simulink model "battery_convertidor_ac_dc_44"  (R2024b)
settings: Solver=FixedStepAuto  StartTime=0.0  StopTime=751  FixedStep=1e-5  RelTol=1e-3
InitFcn:
  | Tint = 1e-5;
  | Ts = 10*Tint;
values from neighbouring files (symbols this model uses):
  C1_filter = 20e-6    (= 2e-05)    [parametros_generales.m]
  I_control = 1    [parametros_generales.m]
  I_control_bat = 5    [parametros_generales.m]
  L_converter = 20e-3    (= 0.02)    [parametros_generales.m]
  Lbat_converter = 1e-5    (= 1e-05)    [parametros_generales.m]
  load_dc = 1000*1000/5    (= 200000)    [parametros_generales.m]
  P_control = 0.01    [parametros_generales.m]
  P_control_bat = 0.7    [parametros_generales.m]
  R = 0.5    [parametros_generales.m]
  R_filter = 0.5    [parametros_generales.m]
  rated_capacitance = 62.5/8    (= 7.8125)    [parametros_generales.m]
  rated_voltage = 144*8    (= 1152)    [parametros_generales.m]
  sample_time_control = 4e-4    (= 0.0004)    [parametros_generales.m]
  voltage_dc_source = 1000    [parametros_generales.m]
undefined symbols (not defined in the file or in its folder): Ion, Lithium
libraries: spsIGBTDiodeLib x24, spsCurrentMeasurementLib x23, spsSeriesRLCBranchLib x20, spsVoltageMeasurementLib x14, dspstat3 x8, spsThreePhaseVIMeasurementLib x8, simulink x7, spsPower3phInstantaneousLib x6, slpidlib x3, spsBatteryLib x2, spsVariableCapacitorLib x1, spsVariableResistorLib x1
(part 1 of 2)
settings Model: Creator=DGY  LastModifiedBy=dagua
settings DataIOCC: SignalLogging=off  DSMLogging=off  ReturnWorkspaceOutputs=off
settings DebuggingCC: UnconnectedInputMsg=warning  UnconnectedOutputMsg=warning  UnconnectedLineMsg=warning
settings ModelReferenceCC: EnableRefExpFcnMdlSchedulingChecks=on
settings RTWCC: GPUComputeCapability=3.5  DLArmComputeVersion=19.05

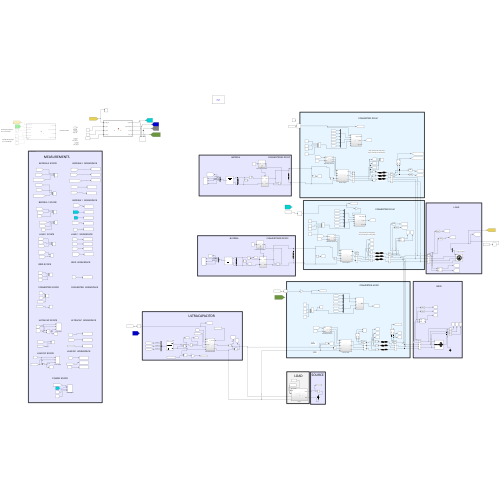
[thumbnail: Simulink's stored preview of the top-level diagram]
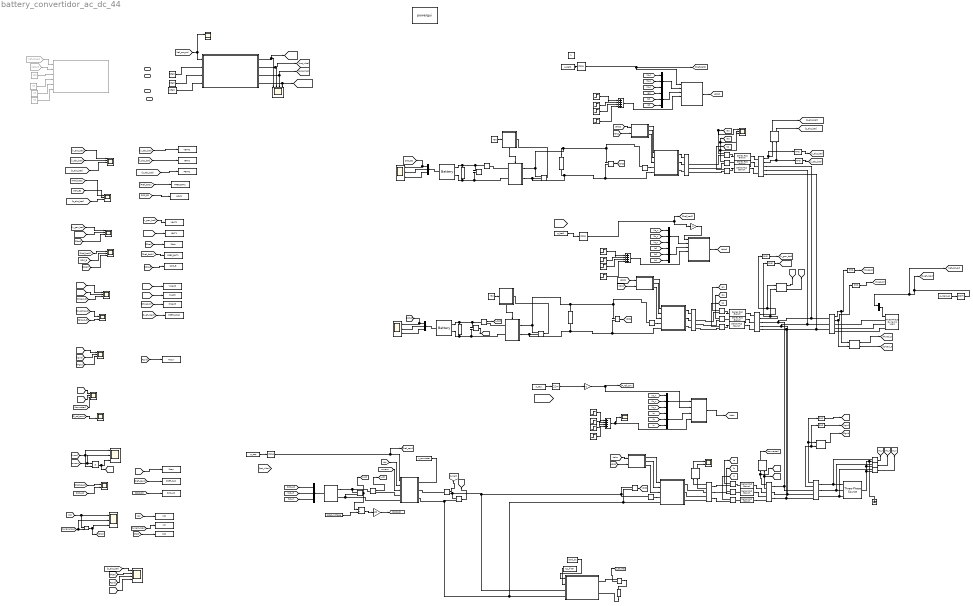
== system battery_convertidor_ac_dc_44 ==
  note: carga en estrella
  note: raiz(3)*Ip/raiz(2)*Vph*raiz(3)/raiz(2)
  note: potencias manuales
  note: i1
  note: Visualización
  note: i2
  note: BATERIA
  note: CONVERTIDOR DC/DC
  note: CONVERTER DC/AC
  note: CONVERTER AC/DC
  note: DC+
  note: DC-
  note: MEASUREMENTS
  note: porcentaje de energia que va a ir a la carga AC
  note: porcentaje de energia que va a ir a la carga DC
  note: raiz(3)*102/raiz(2)*327*raiz(3)/raiz(2)
  note: SOURCE
  note: 35kw
  note: ULTRACAPACITOR
  note: 7s1p
  note: LOAD
  note: 1154
  note: raiz(3)*Ip/raiz(2)*Vph*raiz(3)/raiz(2)
  note: CONVERTIDOR DC/DC
  note: BATERIA
  note: raiz(3)*102/raiz(2)*327*raiz(3)/raiz(2)
  note: CONVERTER DC/AC
  note: BATERIA 2 SCOPE
  note: BATERIA 2 WORKSPACE
  note: BATERIA 1 SCOPE
  note: BATERIA 1 WORKSPACE
  note: GRID SCOPE
  note: GRID WORKSPACE
  note: LOAD
  note: GRID
  note: LOAD 1 WORKSPACE
  note: LOAD 1 SCOPE
  note: ULTRACAP WORKSPACE
  note: ULTRACAP SCOPE
  note: CONVERTER SCOPE
  note: CONVERTER WORKSPACE
  note: LOAD DC WORKSPACE
  note: LOAD DC SCOPE
  note: POWER SCOPE
  Pref_Bat : Inport
  Pref_Ultr : Inport  Port=2
  Pref_smes : Inport  Port=3
  Pref_ac_dc : Inport  Port=4
  Battery : spsBatteryLib/Battery  BatType=Lithium-Ion  NomV=Nominal_voltage  NomQ=Rated_capacity  SOC=initial_state_of_charge  Batt_Tr=battery_time  PresetModel=on  MaxQ=1000  MinV=384  FullV=595.9614  Dis_rate=434.7826  R=0.00512  Normal_OP=904.3478  expZone="[553.1576      49.13043]"
      settings: LibrarySourceBlock=electricdrivelib/Extra Sources/Battery
  Battery1 : spsBatteryLib/Battery  BatType=Lithium-Ion  NomV=Nominal_voltage  NomQ=Rated_capacity  SOC=initial_state_of_charge  Batt_Tr=battery_time  PresetModel=on  MaxQ=1000  MinV=384  FullV=595.9614  Dis_rate=434.7826  R=0.00512  Normal_OP=904.3478  expZone="[553.1576      49.13043]"
      settings: LibrarySourceBlock=electricdrivelib/Extra Sources/Battery
  Bus Selector : BusSelector  OutputSignals=SOC (%),Current (A),Voltage (V)
  Bus Selector1 : BusSelector  OutputSignals=SOC (%),Current (A),Voltage (V)
  Bus Selector2 : BusSelector  OutputSignals=SOC %,Voltage V,Current I
  Carga : Subsystem
  Constant : Constant
  Constant1 : Constant  Value=C1_filter
  Constant10 : Constant  Value=25e3
  Constant13 : Constant  Value=25e3
  Constant15 : Constant  Value=83e3
  Constant16 : Constant  Commented=on  Value=33
  Constant17 : Constant  Commented=on  Value=100
  Constant2 : Constant  Value=750
  Constant3 : Constant  Value=750
  Constant4 : Constant  Value=load_dc
  Constant5 : Constant  Value=rated_voltage
  Constant6 : Constant  Value=L_converter
  Constant8 : Constant  Commented=on  Value=33
  Constant9 : Constant  Commented=on  Value=33
  Control del convertidor1 : Subsystem
      settings: PortSchema="{\"entries\":[{\"content\":{\"sides\":[{\"content\":{\"connectorIds\":[\"In1\"]},\"type\":\"ConnectorPlacement.EquallySpacedRectSide\",\"uuid\":\"952f4d9f-85a3-4809-ab80-f95b4e630059\"},{\"content\":{\"connectorIds\":[\"In2\"],\"side\":\"RIGHT\"},\"type\":\"ConnectorPlacement.EquallySpacedRectSide\",\"uuid\":\"24c0a236-3f22-4c40-86cc-925551a19bc9\"},{\"content\":{\"side\":\"TOP\"},\"type\":\"ConnectorPlacement.EquallySpacedRectSide\",\"uuid\":\"1a366aec-943f-41ae-ba47-6c948c084703\"},{\"content\":{\"connectorIds\":[\"Out1\"],\"side\":\"BOTTOM\"},\"type\":\"ConnectorPlacement.EquallySpacedRectSide\",\"uuid\":\"781da9ee-8b6b-417d-a56c-b699191914ae\"}]},\"type\":\"ConnectorPlacement.EquallySpacedConnector\",\"uuid\":\"c6d9e875-0dde-4ffd-9bd0-64114f723d5e\"}],\"packageUris\":[\"http://schema.mathworks.com/mf0/Connector/R2020b\"],\"version\":\"1.0\"}"
  Control del convertidor2 : Subsystem
      settings: PortSchema="{\"entries\":[{\"content\":{\"sides\":[{\"content\":{\"connectorIds\":[\"In1\"]},\"type\":\"ConnectorPlacement.EquallySpacedRectSide\",\"uuid\":\"952f4d9f-85a3-4809-ab80-f95b4e630059\"},{\"content\":{\"connectorIds\":[\"In2\"],\"side\":\"RIGHT\"},\"type\":\"ConnectorPlacement.EquallySpacedRectSide\",\"uuid\":\"24c0a236-3f22-4c40-86cc-925551a19bc9\"},{\"content\":{\"side\":\"TOP\"},\"type\":\"ConnectorPlacement.EquallySpacedRectSide\",\"uuid\":\"1a366aec-943f-41ae-ba47-6c948c084703\"},{\"content\":{\"connectorIds\":[\"Out1\"],\"side\":\"BOTTOM\"},\"type\":\"ConnectorPlacement.EquallySpacedRectSide\",\"uuid\":\"781da9ee-8b6b-417d-a56c-b699191914ae\"}]},\"type\":\"ConnectorPlacement.EquallySpacedConnector\",\"uuid\":\"c6d9e875-0dde-4ffd-9bd0-64114f723d5e\"}],\"packageUris\":[\"http://schema.mathworks.com/mf0/Connector/R2020b\"],\"version\":\"1.0\"}"
  Current Measurement{,1..16} (17 alike) : spsCurrentMeasurementLib/Current Measurement  PhasorSimulation=off  OutputType=Complex  PSBequivalent=0
  DC Voltage Source1 : spsDCVoltageSourceLib/DC Voltage Source  Amplitude=voltage_dc_source  Measurements=None
  Divide1 : Product  Inputs=*/
  From Workspace : FromWorkspace  VariableName=p_bat1
  From Workspace1 : FromWorkspace  VariableName=p_cap
  From Workspace2 : FromWorkspace  VariableName=p_cap
  From Workspace3 : FromWorkspace  VariableName=p_load_ac
  From Workspace4 : FromWorkspace  VariableName=p_bat2
  From43 : From  Commented=on  GotoTag=ref_pot_ac
  From55 : From  Commented=on  GotoTag=refpot
  Gain1 : Gain  Gain=-1
  Gain2 : Gain  Gain=-1
  Gain3 : Gain  Gain=100
  Ground : spsGroundLib/Ground  LConnTagsString=a
  MATLAB Function : MATLAB Function  Commented=on  TreatAsAtomicUnit=on
  MATLAB Function1 : MATLAB Function  TreatAsAtomicUnit=on
  Modulación puente H1 : Subsystem
  Modulación puente H2 : Subsystem
  Modulación puente H3 : Subsystem
  Mux{1..4,12..13} (6 alike) : Mux  Inputs=3
  Mux17 : Mux  Inputs=2
  Power (3ph, Instantaneous){,2..5,7} (6 alike) : spsPower3phInstantaneousLib/Power (3ph, Instantaneous)
  Product2 : Product
  Product4 : Product
  Puente H 3pha : Subsystem
  Puente H 3pha1 : Subsystem
  Puente H 3pha2 : Subsystem
  RMS{,1..7} (8 alike) : dspstat3/RMS  run=off  directionMode=Each column  dimension=1  InputProcessing=Columns as channels (frame based)  reset_popup=None
  Scope{,1,15,21,41} (5 alike) : Scope  NumInputPorts=2
  Scope{2..3,5,7..8,12,23} (7 alike) : Scope  NumInputPorts=3
  Scope{6,14,19..20} (4 alike) : Scope  NumInputPorts=4
  Scope9 : Scope
  Series RLC Branch{1..4,7..8,11..13} (9 alike) : spsSeriesRLCBranchLib/Series RLC Branch  LConnTagsString=__new0  RConnTagsString=__new0  BranchType=RL  Resistance=0.2  Inductance=5e-3  SetiL0=off  InitialCurrent=0  Capacitance=1e-6  Setx0=off  InitialVoltage=0  Measurements=None
  Series RLC Branch10 : spsSeriesRLCBranchLib/Series RLC Branch  LConnTagsString=__new0  RConnTagsString=__new0  BranchType=RC  Resistance=0.001  Inductance=1e-3  SetiL0=off  InitialCurrent=0  Capacitance=1e-2  Setx0=on  InitialVoltage=512  Measurements=None
  Series RLC Branch5 : spsSeriesRLCBranchLib/Series RLC Branch  LConnTagsString=__new0  RConnTagsString=__new0  BranchType=C  Resistance=0.2  Inductance=1e-3  SetiL0=off  InitialCurrent=0  Capacitance=0.15  Setx0=on  InitialVoltage=600  Measurements=None
  Series RLC Branch6 : spsSeriesRLCBranchLib/Series RLC Branch  LConnTagsString=__new0  RConnTagsString=__new0  BranchType=RC  Resistance=0.001  Inductance=1e-3  SetiL0=off  InitialCurrent=0  Capacitance=1e-2  Setx0=on  InitialVoltage=512  Measurements=None
  Series RLC Branch9 : spsSeriesRLCBranchLib/Series RLC Branch  LConnTagsString=__new0  RConnTagsString=__new0  BranchType=C  Resistance=0.2  Inductance=1e-3  SetiL0=off  InitialCurrent=0  Capacitance=0.15  Setx0=on  InitialVoltage=600  Measurements=None
  Step12 : Step  Time=0.1  Before=-1.5e3  After=-2e3  SampleTime=0
  Step16 : Step  Time=0.2  After=-1e3  SampleTime=0
  Step17 : Step  Time=0.1  Before=-1.5e3  After=-2e3  SampleTime=0
  Step18 : Step  Time=0.2  After=-1e3  SampleTime=0
  Step19 : Step  Time=0.3  After=-1e3  SampleTime=0
  Step20 : Step  Time=0.4  After=-1e3  SampleTime=0
  Step21 : Step  Time=0.3  After=-1e3  SampleTime=0
  Step22 : Step  Time=0.4  After=-1e3  SampleTime=0
  Step6 : Step  Time=0.15  Before=1.5e3  After=2e3  SampleTime=0
  Step7 : Step  Time=0.3  After=1e3  SampleTime=0
  Step8 : Step  Time=0.45  After=1e3  SampleTime=0
  Step9 : Step  After=1e3  SampleTime=0
  "Subs switched model " : Subsystem
      settings: PortSchema="{\"entries\":[{\"content\":{\"sides\":[{\"content\":{\"connectorIds\":[\"In1\",\"In2\",\"In3\",\"LConn1\",\"LConn2\"]},\"type\":\"ConnectorPlacement.EquallySpacedRectSide\",\"uuid\":\"c251221c-47f6-421c-a2d7-5bbfba4f112f\"},{\"content\":{\"connectorIds\":[\"In4\",\"RConn1\",\"RConn2\"],\"side\":\"RIGHT\"},\"type\":\"ConnectorPlacement.EquallySpacedRectSide\",\"uuid\":\"04a66283-5a4b-4f04-b1e9-633aa9198ece\"},{\"content\":{\"side\":\"TOP\"},\"type\":\"ConnectorPlacement.EquallySpacedRectSide\",\"uuid\":\"bb199fa0-295e-40b6-9755-cc304ea24fe5\"}]},\"type\":\"ConnectorPlacement.EquallySpacedConnector\",\"uuid\":\"0b09f002-5912-488f-a17f-ab220b7325f4\"}],\"packageUris\":[\"http://schema.mathworks.com/mf0/Connector/R2020b\"],\"version\":\"1.0\"}"
  Subsystem : Subsystem
  Subsystem1 : Subsystem
  Subsystem2 : Subsystem
  Subsystem3 : Subsystem
      settings: PortSchema="{\"entries\":[{\"content\":{\"sides\":[{\"content\":{\"connectorIds\":[\"LConn1\",\"LConn2\"]},\"type\":\"ConnectorPlacement.EquallySpacedRectSide\",\"uuid\":\"7a980847-0fd3-4a52-ae22-59cd2a1ed559\"},{\"content\":{\"connectorIds\":[\"RConn1\",\"RConn2\"],\"side\":\"RIGHT\"},\"type\":\"ConnectorPlacement.EquallySpacedRectSide\",\"uuid\":\"85effeeb-73a6-4b0a-b51b-5eb0082317ff\"},{\"content\":{\"connectorIds\":[\"In1\"],\"side\":\"TOP\"},\"type\":\"ConnectorPlacement.EquallySpacedRectSide\",\"uuid\":\"eb55fae0-79ad-414f-ab96-49c332138803\"},{\"content\":{\"side\":\"BOTTOM\"},\"type\":\"ConnectorPlacement.EquallySpacedRectSide\",\"uuid\":\"1fd972ff-419a-4657-8ea4-57d89be2b868\"}]},\"type\":\"ConnectorPlacement.EquallySpacedConnector\",\"uuid\":\"1807473d-fd42-44e0-a7e4-668a7bf21429\"}],\"packageUris\":[\"http://schema.mathworks.com/mf0/Connector/R2020b\"],\"version\":\"1.0\"}"
  Subsystem4 : Subsystem
      settings: PortSchema="{\"entries\":[{\"content\":{\"sides\":[{\"content\":{\"connectorIds\":[\"LConn1\",\"LConn2\"]},\"type\":\"ConnectorPlacement.EquallySpacedRectSide\",\"uuid\":\"7a980847-0fd3-4a52-ae22-59cd2a1ed559\"},{\"content\":{\"connectorIds\":[\"RConn1\",\"RConn2\"],\"side\":\"RIGHT\"},\"type\":\"ConnectorPlacement.EquallySpacedRectSide\",\"uuid\":\"85effeeb-73a6-4b0a-b51b-5eb0082317ff\"},{\"content\":{\"connectorIds\":[\"In1\"],\"side\":\"TOP\"},\"type\":\"ConnectorPlacement.EquallySpacedRectSide\",\"uuid\":\"eb55fae0-79ad-414f-ab96-49c332138803\"},{\"content\":{\"side\":\"BOTTOM\"},\"type\":\"ConnectorPlacement.EquallySpacedRectSide\",\"uuid\":\"1fd972ff-419a-4657-8ea4-57d89be2b868\"}]},\"type\":\"ConnectorPlacement.EquallySpacedConnector\",\"uuid\":\"1807473d-fd42-44e0-a7e4-668a7bf21429\"}],\"packageUris\":[\"http://schema.mathworks.com/mf0/Connector/R2020b\"],\"version\":\"1.0\"}"
  Sum1 : Sum  Inputs=|++++
  Sum2 : Sum  Inputs=|++++
  Sum3 : Sum  Inputs=|++++
  Supercapacitor2 : spsSupercapacitorLib/Supercapacitor  C=rated_capacitance  Rdc=equivalent_dc_series  Voltage=rated_voltage  Ns=1  Np=1  Vinit=initial_voltage  Temp=temp  Nc=1  r=1e-9  epsilon=6.0208e-10  Ioc=10  Vself="[48  47.8  47.06  44.65]"
      settings: LibrarySourceBlock=electricdrivelib/Extra Sources/Supercapacitor
  Three-Phase Dynamic Load1 : spsThreePhaseDynamicLoadLib/Three-Phase Dynamic Load  NominalVoltage=[ 400 50 ]  ActiveReactivePowers=[50e3 0]  PositiveSequence=[0.994 -11.8]  ExternalControl=on  NpNq=[1.3 2]  TimeConstants="[0  0  0  0]"  MinimumVoltage=0.7  Tfilter=1e-4  LoadFlowParameters=[4,0,0,0,0]
      settings: LibrarySourceBlock=|
      | sps_lib/Passives/Three-Phase
      | Dynamic Load
  Three-Phase V-I Measurement1 : spsThreePhaseVIMeasurementLib/Three-Phase V-I Measurement  VoltageMeasurement=phase-to-phase  SetLabelV=off  LabelV=Vabc  Vpu=off  VpuLL=off  CurrentMeasurement=yes  SetLabelI=off  LabelI=Iabc  Ipu=off  Pbase=100e6  Vbase=500e3  OutputType=Complex  PhasorSimulation=off  PSBequivalent=0
  Three-Phase V-I Measurement{2..4,6..7} (5 alike) : spsThreePhaseVIMeasurementLib/Three-Phase V-I Measurement  VoltageMeasurement=phase-to-ground  SetLabelV=off  LabelV=Vabc  Vpu=off  VpuLL=off  CurrentMeasurement=yes  SetLabelI=off  LabelI=Iabc  Ipu=off  Pbase=100e6  Vbase=500e3  OutputType=Complex  PhasorSimulation=off  PSBequivalent=0
  Three-Phase V-I Measurement5 : spsThreePhaseVIMeasurementLib/Three-Phase V-I Measurement  VoltageMeasurement=phase-to-phase  SetLabelV=off  LabelV=Vabc  Vpu=off  VpuLL=off  CurrentMeasurement=yes  SetLabelI=off  LabelI=Iabc  Ipu=off  Pbase=100e6  Vbase=500e3  OutputType=Complex  PhasorSimulation=off  PSBequivalent=0
  Three-Phase V-I Measurement9 : spsThreePhaseVIMeasurementLib/Three-Phase V-I Measurement  VoltageMeasurement=phase-to-phase  SetLabelV=off  LabelV=Vabc  Vpu=off  VpuLL=off  CurrentMeasurement=yes  SetLabelI=off  LabelI=Iabc  Ipu=off  Pbase=100e6  Vbase=500e3  OutputType=Complex  PhasorSimulation=off  PSBequivalent=0
  Three-Phase Source : spsThreePhaseSourceLib/Three-Phase Source  InternalConnection=Yn  VoltagePhases=off  Voltage=400  PhaseAngle=0  Voltage_phases=[25e3 25e3 25e3]/sqrt(3)  PhaseAngles_phases=[0 -120 +120]  Frequency=50  NonIdealSource=off  SpecifyImpedance=off  Resistance=0.8929  Inductance=16.58e-3  ShortCircuitLevel=100e6  BaseVoltage=25e3  XRratio=7  BusType=PV  Pref=20e3  Qref=0  Prefabc=[10e3, 10e3, 10e3]  Qrefabc=[0, 0, 0]  Qmin=-inf  Qmax=inf
  To Workspace : ToWorkspace  VariableName=PBAT2  SaveFormat=Timeseries  SampleTime=0.1
  To Workspace1 : ToWorkspace  VariableName=VBAT2  SaveFormat=Timeseries  SampleTime=0.1
  To Workspace10 : ToWorkspace  VariableName=Vdc  SaveFormat=Timeseries  SampleTime=0.1
  To Workspace11 : ToWorkspace  VariableName=SOC_B  SaveFormat=Timeseries  SampleTime=0.1
  To Workspace12 : ToWorkspace  VariableName=IBAT2  SaveFormat=Timeseries  SampleTime=0.1
  To Workspace15 : ToWorkspace  VariableName=VBAT1  SaveFormat=Timeseries  SampleTime=0.1
  To Workspace16 : ToWorkspace  VariableName=IBAT1  SaveFormat=Timeseries  SampleTime=0.1
  To Workspace17 : ToWorkspace  VariableName=SOC2  SaveFormat=Timeseries  SampleTime=0.1
  To Workspace18 : ToWorkspace  VariableName=SOC_UC  SaveFormat=Timeseries  SampleTime=0.1
  To Workspace19 : ToWorkspace  VariableName=PREF_BAT2  SaveFormat=Timeseries  SampleTime=0.1
  To Workspace2 : ToWorkspace  VariableName=Pbat  SaveFormat=Timeseries  SampleTime=0.1
  To Workspace20 : ToWorkspace  VariableName=PREF_BAT1  SaveFormat=Timeseries  SampleTime=0.1
  To Workspace21 : ToWorkspace  VariableName=PREF_CAP  SaveFormat=Timeseries  SampleTime=0.1
  To Workspace23 : ToWorkspace  VariableName=PREF_LOAD  SaveFormat=Timeseries  SampleTime=0.1
  To Workspace3 : ToWorkspace  VariableName=Psour  SaveFormat=Timeseries  SampleTime=0.1
  To Workspace4 : ToWorkspace  VariableName=Pcap  SaveFormat=Timeseries  SampleTime=0.1
  To Workspace5 : ToWorkspace  VariableName=Pdc  SaveFormat=Timeseries  SampleTime=0.1
  To Workspace6 : ToWorkspace  VariableName=Vload3  SaveFormat=Timeseries  SampleTime=0.1
  To Workspace7 : ToWorkspace  VariableName=Pload3  SaveFormat=Timeseries  SampleTime=0.1
  To Workspace8 : ToWorkspace  VariableName=Iload3  SaveFormat=Timeseries  SampleTime=0.1
  To Workspace9 : ToWorkspace  VariableName=Idc  SaveFormat=Timeseries  SampleTime=0.1
  Voltage Measurement{1..12} (12 alike) : spsVoltageMeasurementLib/Voltage Measurement  PhasorSimulation=off  OutputType=Complex  PSBequivalent=0
  Zero-Order Hold{,1..4} (5 alike) : ZeroOrderHold  SampleTime=0.5
  currentvoltaje1 : Scope  NumInputPorts=3
  currentvoltaje2 : Scope  NumInputPorts=3
  currentvoltaje3 : Scope  NumInputPorts=4
  powergui : spspowerguiLib/powergui  Priority=1  SimulationMode=Discrete  SampleTime=1e-5  frequency=60  Iterations=50  frequencyindice=0  Pbase=100e6  ErrMax=1e-4  UnitsV=kV  UnitsW=MW  buscounter=0  FunctionMessages=off  echomessages=off  EnableUseOfTLC=off  CurrentSourceSwitches=off  DisableSnubberDevices=off  DisableRonSwitches=off  DisableVfSwitches=off  DisplayEquations=off  AutomaticDiscreteSolvers=off  SolverType=Tustin/Backward Euler (TBE)  Interpol=off  ExternalGateDelay=off  methode=off  Ts=100  x0status=blocks  SPID=on  SwTol=0  HookPort=off  NonlinearTolerance=1e-4  nMaxIteration=100  ContinueOnMaxIteration=off  RestoreLinks=warning  ResistiveCurrentMeasurement=off  Frange=[0:2:500]  Ylog=off  Xlog=on  ShowGrid=off  save=off  variable=ZData  structure=0  ZoomFFT=off  StartTime=0.0  cycles=1  DisplayStyle=1  fundamental=60  FreqAxis=off  MaxFrequency=1000  frequencyindicesteady=1  RmsSteady=1  display=off
  tag scope: I_UC=global, Ia1=global, Ia2=global, Ia=global, Ib1=global, Ib2=global, Ib=global, Ic1=global, Ic2=global, Ic=global, SOC_B2=global, SOC_B=global, SOC_UC=global, Uabc1=global, Uabc2=global, Uabc=global, VDC0=global, VDC1=global, VDC2=global, V_UC=global, Va_n=global, Vb_n=global, Vc_n=global, current=global
  wires:
  Step9/1 -> Sum1/4
  Current Measurement2/1 -> [Ic]
  [Ib] -> Mux4/2
  Current Measurement/1 -> [Ia]
  Step8/1 -> Sum1/3
  [Vb_n] -> Mux3/2
  Voltage Measurement8/1 -> [V_bat]
  Battery/1 -> Bus Selector/1
  Modulación puente H1/1(Sa) -> Puente H 3pha/1(Sa)
  Constant3/1 -> Control del convertidor1/1(V_ref)
  Voltage Measurement4/1 -> [Va_n]
  [Vc_n] -> Mux3/3
  Bus Selector/2 -> Scope23/2  "<Current (A)>"
  Voltage Measurement6/1 -> [Vc_n]
  Modulación puente H1/2(Sb) -> Puente H 3pha/2(Sb)
  Current Measurement1/1 -> [Ib]
  Voltage Measurement9/1 -> Control del convertidor1/2(Vs)
  [Ia] -> Mux4/1
  [Uabc] -> Modulación puente H1/1(Uabc)
  Step6/1 -> Sum1/1
  Bus Selector/1 -> [SOC_B], Scope23/1  "<SOC (%)>"
  [Ic] -> Mux4/3
  Step7/1 -> Sum1/2
  Three-Phase V-I Measurement1/2 -> "Power (3ph, Instantaneous)3"/2  "Iabc"
  [Va_n] -> Mux3/1
  Current Measurement3/1 -> [I_bat]
  Three-Phase V-I Measurement1/1 -> "Power (3ph, Instantaneous)3"/1  "Vabc"
  Sum1/1 -> Subsystem2/4(In4), Scope9/1
  [VDC0] -> Modulación puente H1/2(VDC)
  Bus Selector/3 -> Scope23/3  "<Voltage (V)>"
  Voltage Measurement5/1 -> [Vb_n]
  Modulación puente H1/3(Sc) -> Puente H 3pha/3(Sc)
  Control del convertidor1/1(Pulse) -> Subsystem3/1(S)
  "Power (3ph, Instantaneous)"/1 -> [Pgrid]
  Three-Phase V-I Measurement4/1 -> RMS4/1, "Power (3ph, Instantaneous)"/1  "Vabc"
  Three-Phase V-I Measurement4/2 -> RMS5/1, "Power (3ph, Instantaneous)"/2
  Modulación puente H2/2(Sb) -> Puente H 3pha1/2(Sb)
  [Ia1] -> Mux13/1
  [Vc_n] -> Mux12/3
  [Uabc1] -> Modulación puente H2/1(Uabc)
  Voltage Measurement3/1 -> [VDC1]
  [Ic1] -> Mux13/3
  [VDC1] -> Modulación puente H2/2(VDC)
  Modulación puente H2/3(Sc) -> Puente H 3pha1/3(Sc)
  [Va_n] -> Mux12/1
  Current Measurement8/1 -> [Ia1]
  Modulación puente H2/1(Sa) -> Puente H 3pha1/1(Sa)
  [Ib1] -> Mux13/2
  Mux17/1 -> Three-Phase Dynamic Load1/1
  Current Measurement11/1 -> [Ib1]
  Current Measurement13/1 -> [Ic1]
  [Vb_n] -> Mux12/2
  Three-Phase V-I Measurement3/1 -> RMS/1, "Power (3ph, Instantaneous)5"/1  "Vabc"
  Three-Phase V-I Measurement3/2 -> "Power (3ph, Instantaneous)5"/2, RMS1/1  "Iabc"
  Step17/1 -> Sum3/1
  Step20/1 -> Sum3/4
  Step19/1 -> Sum3/3
  Step18/1 -> Sum3/2
  "Power (3ph, Instantaneous)2"/1 -> [Pbat]
  Three-Phase V-I Measurement2/1 -> "Power (3ph, Instantaneous)2"/1, RMS2/1  "Vabc"
  Three-Phase V-I Measurement2/2 -> RMS3/1, "Power (3ph, Instantaneous)2"/2  "Iabc"
  "Power (3ph, Instantaneous)3"/1 -> Scope41/1
  "Power (3ph, Instantaneous)3"/2 -> Scope41/2
  "Power (3ph, Instantaneous)4"/1 -> [converter]
  Three-Phase V-I Measurement6/1 -> [vabc_c], "Power (3ph, Instantaneous)4"/1  "Vabc"
  Three-Phase V-I Measurement6/2 -> [iabc_c], "Power (3ph, Instantaneous)4"/2  "Iabc"
  [Pbat] -> To Workspace2/1
  [p_cap] -> To Workspace4/1
  [Pdc] -> To Workspace5/1
  [Pload_3] -> To Workspace7/1
  [Vload_3] -> To Workspace6/1
  [Iload_3] -> To Workspace8/1
  [Current_load] -> To Workspace9/1
  [Vdc] -> To Workspace10/1
  [SOC_B] -> To Workspace11/1
  Mux12/1 -> Subsystem/2(In2)
  Mux13/1 -> Subsystem/3(In3)
  Sum3/1 -> Subsystem/4(In4)
  Subsystem/2(Uabc) -> [Uabc1]
  Mux3/1 -> Subsystem2/1(In1)
  Mux4/1 -> Subsystem2/3(In3)
  Subsystem2/1(Uabc) -> [Uabc]
  Gain2/1 -> Subsystem2/2(In2), [P_ref_conv]
  Zero-Order Hold/1 -> [Pref_bat1], Gain1/1
  Gain1/1 -> Subsystem/1(In1)
  Constant16/1 -> MATLAB Function/6(Per_red)
  From43/1 -> MATLAB Function/1(P_carga_ac)
  Constant8/1 -> MATLAB Function/4(Per_ultra)
  Constant9/1 -> MATLAB Function/5(Per_smes)
  From55/1 -> MATLAB Function/2(P_carga_dc)
  Constant17/1 -> MATLAB Function/3(Per_batt)
  Zero-Order Hold2/1 -> Mux17/1, [ref_pot_ac], [P_ref_load]
  MATLAB Function1/1(P_bateria) -> Scope14/1, [pot_bateria]
  MATLAB Function1/2(P_ultracapacitor) -> [pot_ultra], Scope14/2
  MATLAB Function1/3(P_smes) -> [pot_smes], Scope14/3
  MATLAB Function1/4(P_ac_dc) -> Scope14/4, [pot_red_externa]
  "Power (3ph, Instantaneous)5"/1 -> [Pload_3]
  [ref_pot_ac] -> Scope1/1, MATLAB Function1/1(P_carga_ac)
  RMS/1 -> [Vload_3]
  RMS1/1 -> [Iload_3]
  Constant15/1 -> MATLAB Function1/2(Per_batt)
  Constant10/1 -> MATLAB Function1/3(Per_ultra)
  Constant13/1 -> MATLAB Function1/4(Per_ac_dc)
  Voltage Measurement1/1 -> [vcon]
  Constant1/1 -> Carga/2(Input)
  Current Measurement4/1 -> [current]
  Current Measurement6/1 -> [I_UC]
  Constant4/1 -> Carga/1(load)  "REF_CARGA"
  Supercapacitor2/1 -> Bus Selector2/1
  Current Measurement5/1 -> [I_Source]
  Bus Selector2/2 -> [UC_V]  "<Voltage V>"
  [Vdc] -> "Subs switched model "/2(Vdc)
  Bus Selector2/1 -> [SOC_UC]  "<SOC %>"
  [current] -> "Subs switched model "/3(Current)
  Bus Selector2/3 -> [UC_I]  "<Current I>"
  Zero-Order Hold1/1 -> [Pref_cap1], "Subs switched model "/1(Pref)
  Constant6/1 -> "Subs switched model "/4(L_converter)
  Voltage Measurement2/1 -> [V_UC], Divide1/1
  Product4/1 -> currentvoltaje1/3, [p_cap]  "P_UC"
  [vcon] -> currentvoltaje1/1, Product4/2  "v_UC2"
  [current] -> currentvoltaje1/2, Product4/1  "i_UC2"
  [Vdc] -> currentvoltaje2/1, Product2/1  "Vdc"
  Product2/1 -> [Pdc], currentvoltaje2/3  "P_dc"
  [Current_load] -> currentvoltaje2/2, Product2/2
  Subsystem1/2(Uabc) -> [Uabc2]
  Modulación puente H3/2(Sb) -> Puente H 3pha2/2(Sb)
  Step21/1 -> Sum2/3
  Modulación puente H3/1(Sa) -> Puente H 3pha2/1(Sa)
  Step16/1 -> Sum2/2
  Mux2/1 -> Subsystem1/3(In3)
  Current Measurement10/1 -> [Ic2]
  [Va_n] -> Mux1/1
  [Vb_n] -> Mux1/2
  Three-Phase V-I Measurement7/2 -> "Power (3ph, Instantaneous)7"/2, RMS7/1  "Iabc"
  [Ib2] -> Mux2/2
  Bus Selector1/1 -> [SOC_B2], Scope3/1  "<SOC (%)>"
  Sum2/1 -> Subsystem1/4(In4)
  Battery1/1 -> Bus Selector1/1
  [Uabc2] -> Modulación puente H3/1(Uabc)
  Current Measurement16/1 -> Scope2/1, [Ia2]
  [Ia2] -> Mux2/1
  [Vc_n] -> Mux1/3
  Voltage Measurement11/1 -> Control del convertidor2/2(Vs)
  [Ic2] -> Mux2/3
  Step12/1 -> Sum2/1
  Bus Selector1/2 -> Scope3/2  "<Current (A)>"
  Current Measurement9/1 -> Scope2/3, [Ib2], Scope2/2
  Three-Phase V-I Measurement7/1 -> "Power (3ph, Instantaneous)7"/1, RMS6/1  "Vabc"
  Bus Selector1/3 -> Scope3/3  "<Voltage (V)>"
  Modulación puente H3/3(Sc) -> Puente H 3pha2/3(Sc)
  Step22/1 -> Sum2/4
  Control del convertidor2/1(Pulse) -> Subsystem4/1(S)
  [VDC2] -> Modulación puente H3/2(VDC)
  Voltage Measurement7/1 -> [VDC2]
  Constant2/1 -> Control del convertidor2/1(V_ref)
  Mux1/1 -> Subsystem1/2(In2)
  Zero-Order Hold4/1 -> [Pref_bat2], Subsystem1/1(In1)
  Zero-Order Hold3/1 -> Gain2/1
  From Workspace3/1 -> Zero-Order Hold2/1
  From Workspace1/1 -> Zero-Order Hold1/1  "ref"
  From Workspace2/1 -> Zero-Order Hold3/1  "ref"
  From Workspace4/1 -> Zero-Order Hold4/1
  From Workspace/1 -> Zero-Order Hold/1
  [v_abs_bat] -> To Workspace1/1
  [i_abs_bat] -> Scope19/2
  [v_abs_bat] -> Scope19/1
  [p_abs_bat] -> To Workspace/1
  [i_abs_bat] -> To Workspace12/1
  RMS6/1 -> [v_abs_bat]
  RMS7/1 -> [i_abs_bat]
  [v_gen_bat] -> Scope20/1
  [i_gen_bat] -> Scope20/2
  [Pbat] -> Scope20/3
  [v_gen_bat] -> To Workspace15/1
  [i_gen_bat] -> To Workspace16/1
  RMS2/1 -> [v_gen_bat]
  RMS3/1 -> [i_gen_bat]
  [SOC_B2] -> To Workspace17/1
  Constant5/1 -> Divide1/2
  [SOCUC] -> To Workspace18/1
  Gain3/1 -> [SOCUC]
  Divide1/1 -> Gain3/1
  Voltage Measurement12/1 -> [VDC0]
  "Power (3ph, Instantaneous)7"/1 -> [p_abs_bat]
  "Power (3ph, Instantaneous)7"/2 -> [q_abs_bat]
  [Pref_bat2] -> To Workspace19/1
  [Pref_bat1] -> To Workspace20/1
  "Power (3ph, Instantaneous)2"/2 -> [qbat]
  "Power (3ph, Instantaneous)5"/2 -> [Qload_3]
  [P_ref_load] -> To Workspace23/1
  RMS4/1 -> [Vgrid]
  RMS5/1 -> [Igrid]
  [Vgrid] -> Scope5/1
  [Igrid] -> Scope5/2
  [Pgrid] -> Scope5/3
  [Pgrid] -> To Workspace3/1
  [Pref_cap1] -> To Workspace21/1
  [Pref_cap1] -> Scope21/1
  [P_ref_conv] -> Scope/2
  [vabc_c] -> Scope8/1
  [iabc_c] -> Scope8/2
  [p_abs_bat] -> Scope19/3
  [Pref_bat2] -> Scope7/1
  [SOC_B2] -> Scope7/2
  [q_abs_bat] -> Scope7/3
  [Pref_bat1] -> Scope12/1
  [SOC_B] -> Scope12/2
  [qbat] -> Scope12/3
  [Vload_3] -> Scope6/1
  [Iload_3] -> Scope6/2
  [Pload_3] -> Scope6/3
  [P_ref_load] -> Scope15/1
  [Qload_3] -> Scope15/2
  [converter] -> Scope8/3
  [SOC_UC] -> Scope21/2  "SOC_UC"
  [p_abs_bat] -> currentvoltaje3/1
  [Pbat] -> currentvoltaje3/2
  [Pgrid] -> currentvoltaje3/3
  [p_cap] -> currentvoltaje3/4
  connections:
  Battery/LConn1 -- Series RLC Branch6/LConn1 -- Current Measurement3/LConn1 -- Voltage Measurement8/LConn1
  Battery/LConn2 -- Series RLC Branch6/RConn1 -- Subsystem3/LConn2 -- Voltage Measurement8/LConn2
  Three-Phase Source/RConn1 -- Voltage Measurement4/LConn1 -- Three-Phase V-I Measurement4/LConn1
  Current Measurement14/RConn1 -- Voltage Measurement3/LConn1 -- Subsystem3/RConn1 -- Voltage Measurement9/LConn1 -- Series RLC Branch5/LConn1
  Voltage Measurement5/LConn2 -- Ground/LConn1 -- Voltage Measurement4/LConn2 -- Voltage Measurement6/LConn2 -- Three-Phase Source/LConn1
  Three-Phase V-I Measurement3/LConn1 -- Three-Phase V-I Measurement7/RConn1 -- Three-Phase V-I Measurement2/RConn1 -- Three-Phase V-I Measurement4/RConn1 -- Three-Phase V-I Measurement6/LConn1
  Subsystem3/LConn1 -- Current Measurement3/RConn1
  Series RLC Branch3/LConn1 -- Current Measurement/LConn1
  Three-Phase V-I Measurement1/RConn1 -- Puente H 3pha/RConn1
  Three-Phase V-I Measurement1/LConn3 -- Current Measurement2/RConn1
  Three-Phase V-I Measurement1/LConn1 -- Current Measurement/RConn1
  Three-Phase V-I Measurement1/RConn2 -- Puente H 3pha/RConn2
  Series RLC Branch2/LConn1 -- Current Measurement2/LConn1
  Three-Phase V-I Measurement1/LConn2 -- Current Measurement1/RConn1
  Three-Phase V-I Measurement1/RConn3 -- Puente H 3pha/RConn3
  Series RLC Branch1/LConn1 -- Current Measurement1/LConn1
  Three-Phase Source/RConn2 -- Voltage Measurement5/LConn1 -- Three-Phase V-I Measurement4/LConn2
  Voltage Measurement6/LConn1 -- Three-Phase Source/RConn3 -- Three-Phase V-I Measurement4/LConn3
  Current Measurement7/LConn1 -- Puente H 3pha/LConn1
  Three-Phase V-I Measurement3/LConn2 -- Three-Phase V-I Measurement7/RConn2 -- Three-Phase V-I Measurement2/RConn2 -- Three-Phase V-I Measurement6/LConn2 -- Three-Phase V-I Measurement4/RConn2
  Voltage Measurement9/LConn2 -- Subsystem3/RConn2 -- Series RLC Branch5/RConn1 -- Voltage Measurement3/LConn2 -- Puente H 3pha1/LConn2
  Three-Phase V-I Measurement3/LConn3 -- Three-Phase V-I Measurement7/RConn3 -- Three-Phase V-I Measurement2/RConn3 -- Three-Phase V-I Measurement6/LConn3 -- Three-Phase V-I Measurement4/RConn3
  Puente H 3pha1/RConn2 -- Three-Phase V-I Measurement5/LConn2
  Current Measurement11/RConn1 -- Three-Phase V-I Measurement5/RConn2
  Current Measurement14/LConn1 -- Puente H 3pha1/LConn1
  Series RLC Branch13/LConn1 -- Current Measurement8/LConn1
  Three-Phase V-I Measurement5/LConn3 -- Puente H 3pha1/RConn3
  Puente H 3pha1/RConn1 -- Three-Phase V-I Measurement5/LConn1
  Current Measurement8/RConn1 -- Three-Phase V-I Measurement5/RConn1
  Series RLC Branch11/LConn1 -- Current Measurement11/LConn1
  Series RLC Branch12/LConn1 -- Current Measurement13/LConn1
  Current Measurement13/RConn1 -- Three-Phase V-I Measurement5/RConn3
  Three-Phase Dynamic Load1/LConn1 -- Three-Phase V-I Measurement3/RConn1
  Three-Phase Dynamic Load1/LConn2 -- Three-Phase V-I Measurement3/RConn2
  Three-Phase Dynamic Load1/LConn3 -- Three-Phase V-I Measurement3/RConn3
  Series RLC Branch13/RConn1 -- Three-Phase V-I Measurement2/LConn1
  Series RLC Branch11/RConn1 -- Three-Phase V-I Measurement2/LConn2
  Series RLC Branch12/RConn1 -- Three-Phase V-I Measurement2/LConn3
  Series RLC Branch3/RConn1 -- Three-Phase V-I Measurement6/RConn1
  Series RLC Branch1/RConn1 -- Three-Phase V-I Measurement6/RConn2
  Series RLC Branch2/RConn1 -- Three-Phase V-I Measurement6/RConn3
  Supercapacitor2/LConn2 -- "Subs switched model "/LConn2 -- Voltage Measurement2/LConn2
  Current Measurement4/RConn1 -- Voltage Measurement1/LConn1 -- Voltage Measurement12/LConn1 -- Current Measurement7/RConn1 -- Carga/LConn1
  Voltage Measurement1/LConn2 -- "Subs switched model "/RConn2 -- Voltage Measurement12/LConn2 -- Puente H 3pha/LConn2 -- Carga/LConn2
  Voltage Measurement2/LConn1 -- Current Measurement6/LConn1 -- Supercapacitor2/LConn1
  DC Voltage Source1/LConn1 -- Carga/RConn2
  "Subs switched model "/LConn1 -- Current Measurement6/RConn1
  Current Measurement5/LConn1 -- DC Voltage Source1/RConn1
  Current Measurement5/RConn1 -- Carga/RConn1
  Current Measurement4/LConn1 -- "Subs switched model "/RConn1
  Puente H 3pha2/LConn2 -- Voltage Measurement11/LConn2 -- Subsystem4/RConn2 -- Series RLC Branch9/RConn1 -- Voltage Measurement7/LConn2
  Voltage Measurement10/LConn2 -- Battery1/LConn2 -- Series RLC Branch10/RConn1 -- Subsystem4/LConn2
  Series RLC Branch9/LConn1 -- Voltage Measurement7/LConn1 -- Current Measurement12/RConn1 -- Subsystem4/RConn1 -- Voltage Measurement11/LConn1
  Voltage Measurement10/LConn1 -- Current Measurement15/LConn1 -- Battery1/LConn1 -- Series RLC Branch10/LConn1
  Puente H 3pha2/RConn1 -- Three-Phase V-I Measurement9/LConn1
  Series RLC Branch8/LConn1 -- Current Measurement16/LConn1
  Current Measurement12/LConn1 -- Puente H 3pha2/LConn1
  Puente H 3pha2/RConn2 -- Three-Phase V-I Measurement9/LConn2
  Series RLC Branch7/RConn1 -- Three-Phase V-I Measurement7/LConn3
  Current Measurement9/RConn1 -- Three-Phase V-I Measurement9/RConn2
  Series RLC Branch4/RConn1 -- Three-Phase V-I Measurement7/LConn2
  Series RLC Branch7/LConn1 -- Current Measurement10/LConn1
  Subsystem4/LConn1 -- Current Measurement15/RConn1
  Series RLC Branch4/LConn1 -- Current Measurement9/LConn1
  Series RLC Branch8/RConn1 -- Three-Phase V-I Measurement7/LConn1
  Current Measurement16/RConn1 -- Three-Phase V-I Measurement9/RConn1
  Three-Phase V-I Measurement9/LConn3 -- Puente H 3pha2/RConn3
  Current Measurement10/RConn1 -- Three-Phase V-I Measurement9/RConn3

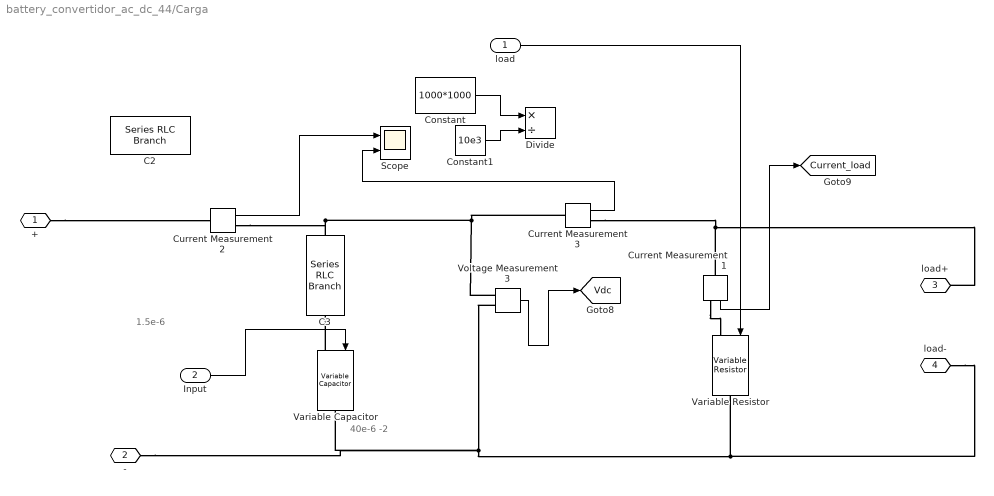
== system battery_convertidor_ac_dc_44/Carga ==
  note: 40e-6 -2
  note: 1.5e-6
  load : Inport
  Input : Inport  Port=2
  C2 : spsSeriesRLCBranchLib/Series RLC Branch  LConnTagsString=__new0  RConnTagsString=__new0  BranchType=R  Resistance=R  Inductance=1e-3  SetiL0=off  InitialCurrent=0  Capacitance=120e-6  Setx0=on  InitialVoltage=1000  Measurements=None
  C3 : spsSeriesRLCBranchLib/Series RLC Branch  LConnTagsString=__new0  RConnTagsString=__new0  BranchType=R  Resistance=R_filter  Inductance=1e-3  SetiL0=off  InitialCurrent=0  Capacitance=120e-6  Setx0=on  InitialVoltage=1000  Measurements=None
  Constant : Constant  Value=1000*1000
  Constant1 : Constant  Value=10e3
  Current Measurement1 : spsCurrentMeasurementLib/Current Measurement  PhasorSimulation=off  OutputType=Complex  PSBequivalent=0
  Current Measurement2 : spsCurrentMeasurementLib/Current Measurement  PhasorSimulation=off  OutputType=Complex  PSBequivalent=0
  Current Measurement3 : spsCurrentMeasurementLib/Current Measurement  PhasorSimulation=off  OutputType=Complex  PSBequivalent=0
  Divide : Product  Inputs=*/
  Scope : Scope  NumInputPorts=2
  Variable Capacitor : spsVariableCapacitorLib/Variable Capacitor  methode=Backward Euler  Cabsmin=1e-9  Initialize=off  vC0=0  C0=1e-6  iC0=2000
  Variable Resistor : spsVariableResistorLib/Variable Resistor  Rabsmin=1e-3
  Voltage Measurement3 : spsVoltageMeasurementLib/Voltage Measurement  PhasorSimulation=off  OutputType=Complex  PSBequivalent=0
  + : PMIOPort  Side=Left
  - : PMIOPort  Port=2  Side=Left
  load+ : PMIOPort  Port=3  Side=Right
  load- : PMIOPort  Port=4  Side=Right
  tag scope: Current_load=global, Vdc=global
  wires:
  Voltage Measurement3/1 -> [Vdc]
  Current Measurement1/1 -> [Current_load]
  Input/1 -> Variable Capacitor/1
  Constant1/1 -> Divide/2
  Constant/1 -> Divide/1
  Current Measurement2/1 -> Scope/1
  Current Measurement3/1 -> Scope/2
  load/1 -> Variable Resistor/1
  connections:
  Voltage Measurement3/LConn2 -- Variable Capacitor/RConn1 -- -/RConn1 -- Variable Resistor/RConn1 -- load-/RConn1
  Voltage Measurement3/LConn1 -- Current Measurement3/LConn1 -- Current Measurement2/RConn1 -- C3/RConn1
  Variable Capacitor/LConn1 -- C3/LConn1
  Current Measurement1/RConn1 -- Variable Resistor/LConn1
  +/RConn1 -- Current Measurement2/LConn1
  Current Measurement1/LConn1 -- Current Measurement3/RConn1 -- load+/RConn1

== system battery_convertidor_ac_dc_44/Control del convertidor1 ==
  note: 0.08 aceptable
  note: 0.15 top
  V_ref : Inport
  Vs : Inport  Port=2
  Constant : Constant
  Divide : Product  Inputs=*/
  PID1 : slpidlib/PID Controller  Controller=PI  Form=Parallel  TimeDomain=Discrete-time  UseExternalTs=off  SampleTime=Ts  IntegratorMethod=Forward Euler  FilterMethod=Forward Euler  ControllerParametersSource=internal  P=P_control_bat  I=I_control_bat  UseKiTs=off  D=0  UseExternalDerivativeSource=off  N=100  UseFilter=on  TunerSelectOption=Transfer Function Based (PID Tuner App)  InitialConditionSource=internal  InitialConditionForIntegrator=0.26  InitialConditionForFilter=0  DifferentiatorICPrevScaledInput=0  ExternalReset=none  TrackingMode=off  Kt=1  LimitOutput=on  SatLimitsSource=internal  UpperSaturationLimit=0.97  LowerSaturationLimit=0  LinearizeAsGain=on  AntiWindupMode=clamping  Kb=1  LimitIntegrator=off  UpperIntegratorSaturationLimit=inf  LowerIntegratorSaturationLimit=-inf  POutMin=[]  POutMax=[]  IOutMin=[]  IOutMax=[]  DOutMin=[]  DOutMax=[]  NOutMin=[]  NOutMax=[]  SumOutMin=[]  SumOutMax=[]  SaturationOutMin=[]  SaturationOutMax=[]  PParamMin=[]  PParamMax=[]  IParamMin=[]  IParamMax=[]  DParamMin=[]  DParamMax=[]  NParamMin=[]  NParamMax=[]  KbParamMin=[]  KbParamMax=[]  KtParamMin=[]  KtParamMax=[]  KbOutMin=[]  KbOutMax=[]  KtOutMin=[]  KtOutMax=[]  IntegratorOutMin=[]  IntegratorOutMax=[]  FilterOutMin=[]  FilterOutMax=[]  SumI1OutMin=[]  SumI1OutMax=[]  SumI2OutMin=[]  SumI2OutMax=[]  SumI3OutMin=[]  SumI3OutMax=[]  SumI4OutMin=[]  SumI4OutMax=[]  SumDOutMin=[]  SumDOutMax=[]  DifferentiatorOutMin=[]  DifferentiatorOutMax=[]  FilterDiffOutCoefMin=[]  FilterDiffOutCoefMax=[]  ReciprocalOutMin=[]  ReciprocalOutMax=[]  SumDenOutMin=[]  SumDenOutMax=[]  SumNumOutMin=[]  SumNumOutMax=[]  DivideOutMin=[]  DivideOutMax=[]  UdiffTsProdOutMin=[]  UdiffTsProdOutMax=[]  NTsProdOutMin=[]  NTsProdOutMax=[]  UintegralTsProdOutMin=[]  UintegralTsProdOutMax=[]  UngainTsProdOutMin=[]  UngainTsProdOutMax=[]  ClampingZeroOutDataTypeStr=Inherit: Inherit via back propagation  ClampingZeroOutMin=[]  ClampingZeroOutMax=[]  FilterDenConstantOutDataTypeStr=Inherit: Inherit via back propagation  FilterDenConstantOutMin=[]  FilterDenConstantOutMax=[]  PCopyOutDataTypeStr=Inherit: Inherit via back propagation  PCopyOutMin=[]  PCopyOutMax=[]  NCopyOutDataTypeStr=Inherit: Inherit via back propagation  NCopyOutMin=[]  NCopyOutMax=[]  IntegratorContinuousStateAttributes=''  IntegratorStateMustResolveToSignalObject=off  IntegratorRTWStateStorageClass=Auto  FilterContinuousStateAttributes=''  FilterStateMustResolveToSignalObject=off  FilterRTWStateStorageClass=Auto  ParallelPVariant=InternalParameters  IdealPVariant=Disabled  IVariant=InternalParameters  DVariant=Disabled  IntegratorVariant=Discrete  SatVariant=Enabled  AWVariant=DiscClampingParallel  PCopyVariant=Disabled  TRVariant=Disabled  FdbkBlocksVariant=Forward  IdealPFdbkVariant=Disabled  SatFdbkVariant=Disabled  DerivativeFilterVariant=Disabled  NVariant=Disabled  NCopyVariant=Disabled_SignalSpec  FilterICVariant=Disabled  IntegratorICVariant=InternalICs  ExternalResetVariant=Disabled  TRSumVariant=Passthrough  SumFdbkVariant=Disabled  SumVariant=Sum_PI  TsampFilterVariant=InternalTs  TsampNgainVariant=Passthrough  TsampIntegralVariant=Disabled_SignalSpec  ExternalSaturationOutDataTypeStr=Inherit: Same as second input  DerivativeSourceVariant=Disabled  PreIntVariant=InternalPreInt
  Relational Operator1 : RelationalOperator  OutDataTypeStr=boolean  InputSameDT=off
  Repeating Sequence2 : simulink/Sources/Repeating Sequence  rep_seq_t=[0 Ts/2 Ts]  rep_seq_y=[0 1 0]
  Scope : Scope  NumInputPorts=3
  Scope1 : Scope  NumInputPorts=3
  Sum7 : Sum  Inputs=|+-
  Pulse : Outport
  wires:
  Sum7/1 -> Scope1/2, PID1/1  "I_B_Actuation"
  Relational Operator1/1 -> Pulse/1, Scope/3  "S2"
  Repeating Sequence2/1 -> Scope/2, Relational Operator1/2
  Constant/1 -> Scope1/1, Sum7/1
  Vs/1 -> Divide/1  "v dc link"
  V_ref/1 -> Divide/2
  Divide/1 -> Sum7/2
  PID1/1 -> Scope1/3, Relational Operator1/1

== system battery_convertidor_ac_dc_44/Control del convertidor2 ==
  note: 0.08 aceptable
  note: 0.15 top
  V_ref : Inport
  Vs : Inport  Port=2
  Constant : Constant
  Divide : Product  Inputs=*/
  PID1 : slpidlib/PID Controller  Controller=PI  Form=Parallel  TimeDomain=Discrete-time  UseExternalTs=off  SampleTime=Ts  IntegratorMethod=Forward Euler  FilterMethod=Forward Euler  ControllerParametersSource=internal  P=P_control_bat  I=I_control_bat  UseKiTs=off  D=0  UseExternalDerivativeSource=off  N=100  UseFilter=on  TunerSelectOption=Transfer Function Based (PID Tuner App)  InitialConditionSource=internal  InitialConditionForIntegrator=0.26  InitialConditionForFilter=0  DifferentiatorICPrevScaledInput=0  ExternalReset=none  TrackingMode=off  Kt=1  LimitOutput=on  SatLimitsSource=internal  UpperSaturationLimit=0.97  LowerSaturationLimit=0  LinearizeAsGain=on  AntiWindupMode=clamping  Kb=1  LimitIntegrator=off  UpperIntegratorSaturationLimit=inf  LowerIntegratorSaturationLimit=-inf  POutMin=[]  POutMax=[]  IOutMin=[]  IOutMax=[]  DOutMin=[]  DOutMax=[]  NOutMin=[]  NOutMax=[]  SumOutMin=[]  SumOutMax=[]  SaturationOutMin=[]  SaturationOutMax=[]  PParamMin=[]  PParamMax=[]  IParamMin=[]  IParamMax=[]  DParamMin=[]  DParamMax=[]  NParamMin=[]  NParamMax=[]  KbParamMin=[]  KbParamMax=[]  KtParamMin=[]  KtParamMax=[]  KbOutMin=[]  KbOutMax=[]  KtOutMin=[]  KtOutMax=[]  IntegratorOutMin=[]  IntegratorOutMax=[]  FilterOutMin=[]  FilterOutMax=[]  SumI1OutMin=[]  SumI1OutMax=[]  SumI2OutMin=[]  SumI2OutMax=[]  SumI3OutMin=[]  SumI3OutMax=[]  SumI4OutMin=[]  SumI4OutMax=[]  SumDOutMin=[]  SumDOutMax=[]  DifferentiatorOutMin=[]  DifferentiatorOutMax=[]  FilterDiffOutCoefMin=[]  FilterDiffOutCoefMax=[]  ReciprocalOutMin=[]  ReciprocalOutMax=[]  SumDenOutMin=[]  SumDenOutMax=[]  SumNumOutMin=[]  SumNumOutMax=[]  DivideOutMin=[]  DivideOutMax=[]  UdiffTsProdOutMin=[]  UdiffTsProdOutMax=[]  NTsProdOutMin=[]  NTsProdOutMax=[]  UintegralTsProdOutMin=[]  UintegralTsProdOutMax=[]  UngainTsProdOutMin=[]  UngainTsProdOutMax=[]  ClampingZeroOutDataTypeStr=Inherit: Inherit via back propagation  ClampingZeroOutMin=[]  ClampingZeroOutMax=[]  FilterDenConstantOutDataTypeStr=Inherit: Inherit via back propagation  FilterDenConstantOutMin=[]  FilterDenConstantOutMax=[]  PCopyOutDataTypeStr=Inherit: Inherit via back propagation  PCopyOutMin=[]  PCopyOutMax=[]  NCopyOutDataTypeStr=Inherit: Inherit via back propagation  NCopyOutMin=[]  NCopyOutMax=[]  IntegratorContinuousStateAttributes=''  IntegratorStateMustResolveToSignalObject=off  IntegratorRTWStateStorageClass=Auto  FilterContinuousStateAttributes=''  FilterStateMustResolveToSignalObject=off  FilterRTWStateStorageClass=Auto  ParallelPVariant=InternalParameters  IdealPVariant=Disabled  IVariant=InternalParameters  DVariant=Disabled  IntegratorVariant=Discrete  SatVariant=Enabled  AWVariant=DiscClampingParallel  PCopyVariant=Disabled  TRVariant=Disabled  FdbkBlocksVariant=Forward  IdealPFdbkVariant=Disabled  SatFdbkVariant=Disabled  DerivativeFilterVariant=Disabled  NVariant=Disabled  NCopyVariant=Disabled_SignalSpec  FilterICVariant=Disabled  IntegratorICVariant=InternalICs  ExternalResetVariant=Disabled  TRSumVariant=Passthrough  SumFdbkVariant=Disabled  SumVariant=Sum_PI  TsampFilterVariant=InternalTs  TsampNgainVariant=Passthrough  TsampIntegralVariant=Disabled_SignalSpec  ExternalSaturationOutDataTypeStr=Inherit: Same as second input  DerivativeSourceVariant=Disabled  PreIntVariant=InternalPreInt
  Relational Operator1 : RelationalOperator  OutDataTypeStr=boolean  InputSameDT=off
  Repeating Sequence2 : simulink/Sources/Repeating Sequence  rep_seq_t=[0 Ts/2 Ts]  rep_seq_y=[0 1 0]
  Scope : Scope  NumInputPorts=3
  Scope1 : Scope  NumInputPorts=3
  Sum7 : Sum  Inputs=|+-
  Pulse : Outport
  wires:
  Sum7/1 -> Scope1/2, PID1/1  "I_B_Actuation"
  Relational Operator1/1 -> Pulse/1, Scope/3  "S2"
  Repeating Sequence2/1 -> Scope/2, Relational Operator1/2
  Constant/1 -> Scope1/1, Sum7/1
  Vs/1 -> Divide/1  "v dc link"
  V_ref/1 -> Divide/2
  Divide/1 -> Sum7/2
  PID1/1 -> Scope1/3, Relational Operator1/1

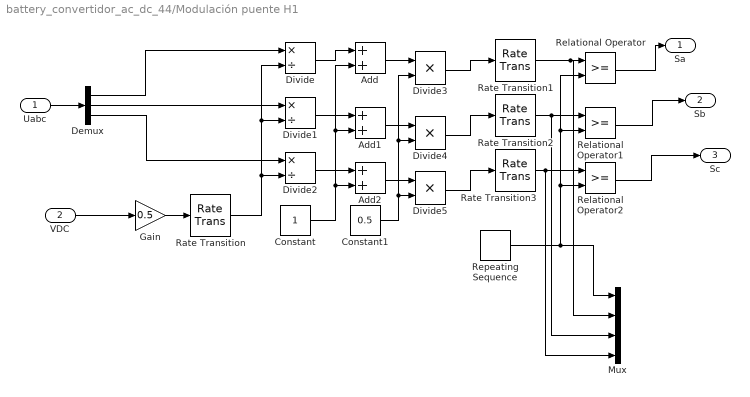
== system battery_convertidor_ac_dc_44/Modulación puente H1 ==
  Uabc : Inport
  VDC : Inport  Port=2
  Add : Sum
  Add1 : Sum
  Add2 : Sum
  Constant : Constant
  Constant1 : Constant  Value=0.5
  Demux : Demux  Outputs=3
  Divide : Product  Inputs=*/
  Divide1 : Product  Inputs=*/
  Divide2 : Product  Inputs=*/
  Divide3 : Product  Inputs=**
  Divide4 : Product  Inputs=**
  Divide5 : Product  Inputs=**
  Gain : Gain  Gain=0.5
  Mux : Mux
  Rate Transition : RateTransition  OutPortSampleTime=Ts
  Rate Transition1 : RateTransition  OutPortSampleTime=Tint
  Rate Transition2 : RateTransition  OutPortSampleTime=Tint
  Rate Transition3 : RateTransition  OutPortSampleTime=Tint
  Relational Operator : RelationalOperator  OutDataTypeStr=boolean  RndMeth=Simplest  InputSameDT=off
  Relational Operator1 : RelationalOperator  OutDataTypeStr=boolean  RndMeth=Simplest  InputSameDT=off
  Relational Operator2 : RelationalOperator  OutDataTypeStr=boolean  RndMeth=Simplest  InputSameDT=off
  Repeating Sequence : simulink/Sources/Repeating Sequence  rep_seq_t=[0 Ts/2 Ts]  rep_seq_y=[0 1 0]
  Sa : Outport
  Sb : Outport  Port=2
  Sc : Outport  Port=3
  wires:
  Demux/3 -> Divide2/1
  Demux/1 -> Divide/1
  Demux/2 -> Divide1/1
  Relational Operator/1 -> Sa/1
  Relational Operator1/1 -> Sb/1
  Relational Operator2/1 -> Sc/1
  Rate Transition/1 -> Divide1/2, Divide/2, Divide2/2
  Divide/1 -> Add/1
  Add/1 -> Divide3/1
  Divide3/1 -> Rate Transition1/1
  Add1/1 -> Divide4/1
  Add2/1 -> Divide5/1
  Divide1/1 -> Add1/1
  Divide4/1 -> Rate Transition2/1
  Divide2/1 -> Add2/1
  Divide5/1 -> Rate Transition3/1
  Constant/1 -> Add2/2, Add1/2, Add/2
  Constant1/1 -> Divide5/2, Divide4/2, Divide3/2
  Uabc/1 -> Demux/1
  Repeating Sequence/1 -> Mux/1, Relational Operator2/2, Relational Operator1/2, Relational Operator/2
  Rate Transition3/1 -> Mux/4, Relational Operator2/1
  Rate Transition2/1 -> Mux/3, Relational Operator1/1
  Rate Transition1/1 -> Mux/2, Relational Operator/1
  Gain/1 -> Rate Transition/1
  VDC/1 -> Gain/1

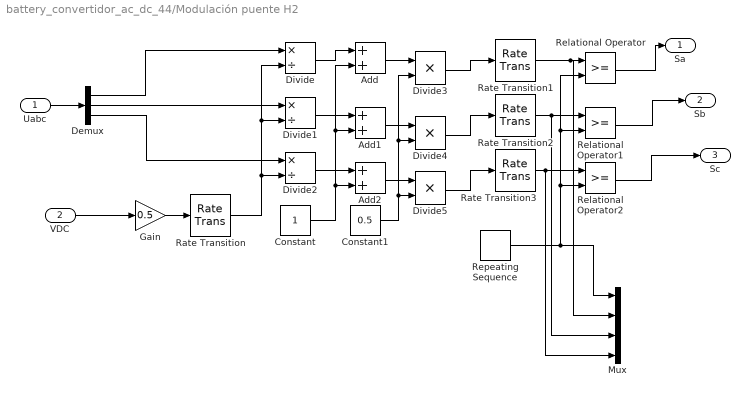
== system battery_convertidor_ac_dc_44/Modulación puente H2 ==
  Uabc : Inport
  VDC : Inport  Port=2
  Add : Sum
  Add1 : Sum
  Add2 : Sum
  Constant : Constant
  Constant1 : Constant  Value=0.5
  Demux : Demux  Outputs=3
  Divide : Product  Inputs=*/
  Divide1 : Product  Inputs=*/
  Divide2 : Product  Inputs=*/
  Divide3 : Product  Inputs=**
  Divide4 : Product  Inputs=**
  Divide5 : Product  Inputs=**
  Gain : Gain  Gain=0.5
  Mux : Mux
  Rate Transition : RateTransition  OutPortSampleTime=Ts
  Rate Transition1 : RateTransition  OutPortSampleTime=Tint
  Rate Transition2 : RateTransition  OutPortSampleTime=Tint
  Rate Transition3 : RateTransition  OutPortSampleTime=Tint
  Relational Operator : RelationalOperator  OutDataTypeStr=boolean  RndMeth=Simplest  InputSameDT=off
  Relational Operator1 : RelationalOperator  OutDataTypeStr=boolean  RndMeth=Simplest  InputSameDT=off
  Relational Operator2 : RelationalOperator  OutDataTypeStr=boolean  RndMeth=Simplest  InputSameDT=off
  Repeating Sequence : simulink/Sources/Repeating Sequence  rep_seq_t=[0 Ts/2 Ts]  rep_seq_y=[0 1 0]
  Sa : Outport
  Sb : Outport  Port=2
  Sc : Outport  Port=3
  wires:
  Demux/3 -> Divide2/1
  Demux/1 -> Divide/1
  Demux/2 -> Divide1/1
  Relational Operator/1 -> Sa/1
  Relational Operator1/1 -> Sb/1
  Relational Operator2/1 -> Sc/1
  Rate Transition/1 -> Divide1/2, Divide/2, Divide2/2
  Divide/1 -> Add/1
  Add/1 -> Divide3/1
  Divide3/1 -> Rate Transition1/1
  Add1/1 -> Divide4/1
  Add2/1 -> Divide5/1
  Divide1/1 -> Add1/1
  Divide4/1 -> Rate Transition2/1
  Divide2/1 -> Add2/1
  Divide5/1 -> Rate Transition3/1
  Constant/1 -> Add2/2, Add1/2, Add/2
  Constant1/1 -> Divide5/2, Divide4/2, Divide3/2
  Uabc/1 -> Demux/1
  Repeating Sequence/1 -> Mux/1, Relational Operator2/2, Relational Operator1/2, Relational Operator/2
  Rate Transition3/1 -> Mux/4, Relational Operator2/1
  Rate Transition2/1 -> Mux/3, Relational Operator1/1
  Rate Transition1/1 -> Mux/2, Relational Operator/1
  Gain/1 -> Rate Transition/1
  VDC/1 -> Gain/1

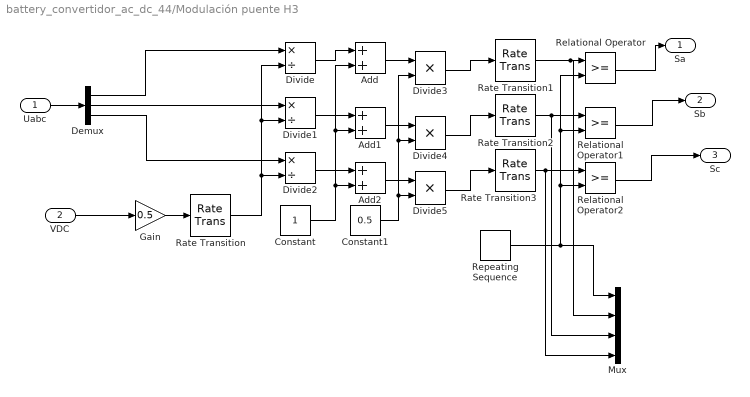
== system battery_convertidor_ac_dc_44/Modulación puente H3 ==
  Uabc : Inport
  VDC : Inport  Port=2
  Add : Sum
  Add1 : Sum
  Add2 : Sum
  Constant : Constant
  Constant1 : Constant  Value=0.5
  Demux : Demux  Outputs=3
  Divide : Product  Inputs=*/
  Divide1 : Product  Inputs=*/
  Divide2 : Product  Inputs=*/
  Divide3 : Product  Inputs=**
  Divide4 : Product  Inputs=**
  Divide5 : Product  Inputs=**
  Gain : Gain  Gain=0.5
  Mux : Mux
  Rate Transition : RateTransition  OutPortSampleTime=Ts
  Rate Transition1 : RateTransition  OutPortSampleTime=Tint
  Rate Transition2 : RateTransition  OutPortSampleTime=Tint
  Rate Transition3 : RateTransition  OutPortSampleTime=Tint
  Relational Operator : RelationalOperator  OutDataTypeStr=boolean  RndMeth=Simplest  InputSameDT=off
  Relational Operator1 : RelationalOperator  OutDataTypeStr=boolean  RndMeth=Simplest  InputSameDT=off
  Relational Operator2 : RelationalOperator  OutDataTypeStr=boolean  RndMeth=Simplest  InputSameDT=off
  Repeating Sequence : simulink/Sources/Repeating Sequence  rep_seq_t=[0 Ts/2 Ts]  rep_seq_y=[0 1 0]
  Sa : Outport
  Sb : Outport  Port=2
  Sc : Outport  Port=3
  wires:
  Demux/3 -> Divide2/1
  Demux/1 -> Divide/1
  Demux/2 -> Divide1/1
  Relational Operator/1 -> Sa/1
  Relational Operator1/1 -> Sb/1
  Relational Operator2/1 -> Sc/1
  Rate Transition/1 -> Divide1/2, Divide/2, Divide2/2
  Divide/1 -> Add/1
  Add/1 -> Divide3/1
  Divide3/1 -> Rate Transition1/1
  Add1/1 -> Divide4/1
  Add2/1 -> Divide5/1
  Divide1/1 -> Add1/1
  Divide4/1 -> Rate Transition2/1
  Divide2/1 -> Add2/1
  Divide5/1 -> Rate Transition3/1
  Constant/1 -> Add2/2, Add1/2, Add/2
  Constant1/1 -> Divide5/2, Divide4/2, Divide3/2
  Uabc/1 -> Demux/1
  Repeating Sequence/1 -> Mux/1, Relational Operator2/2, Relational Operator1/2, Relational Operator/2
  Rate Transition3/1 -> Mux/4, Relational Operator2/1
  Rate Transition2/1 -> Mux/3, Relational Operator1/1
  Rate Transition1/1 -> Mux/2, Relational Operator/1
  Gain/1 -> Rate Transition/1
  VDC/1 -> Gain/1
